simulink library "aerolibwind2"  (Simulink 6.0)
values from neighbouring files (symbols this model uses):
  s = aeroliblist    [asbhelp.m]
undefined symbols (not defined in the file or in its folder): F, ft, Light, m, MIL
libraries: aerolibconvert x11, aerolibwind2 x10, simulink x5, aerolibwindfilters x4, aerolibutil x2
settings Model: Creator=sgage  LastModifiedBy=sgage  ExtModeAutoUpdateStatusClock=off

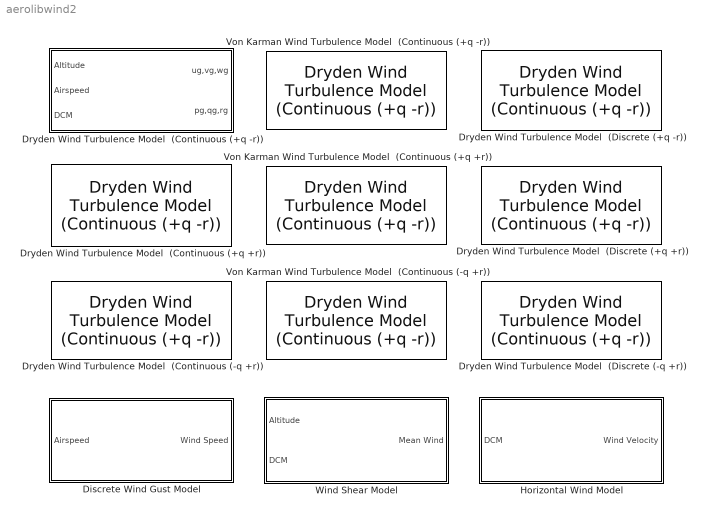
== system aerolibwind2 ==
  Discrete Wind Gust Model : Subsystem  mask(Discrete Wind Gust Model){units=Metric (MKS), Gx=on, Gy=on, Gz=on, t_0=5, d_m=[120 120 80], v_m=[3.5 3.5 3.0]}
      mask prompts: Gx "Gust in u-axis"; Gy "Gust in v-axis"; Gz "Gust in w-axis"; t_0 "Gust start time (sec):"; d_m "Gust length [dx dy dz] (m):"; v_m "Gust amplitude [ug vg wg] (m/s):"
      mask help: Generate a discrete wind gust. The gust profile takes the '1-cosine' form.
      mask init:
      | [ports] = aeroicon('aeroblkwindgust2','icon');
      | [x y highstr lowstr maxy miny] = aeroimage('wind','Discrete Gust');
      mask Help: web(asbhelp);
      mask StyleString: popup(Metric (MKS)|English (Velocity in ft/s)|English (Velocity in kts)),checkbox,checkbox,checkbox,edit,edit,edit
      mask Display:
      | port_label(ports(1).type,ports(1).port,ports(1).txt,'texmode','on');
      | port_label(ports(2).type,ports(2).port,ports(2).txt,'texmode','on');
      | plot(x,y)
      | text(0.5,miny-0.05,lowstr,'HorizontalAlignment','center')
  Dryden Wind Turbulence Model  (Continuous (+q +r)) : aerolibwind2/Dryden Wind Turbulence Model  (Continuous (+q -r))  units=Metric (MKS)  spec=MIL-F-8785C  model=Continuous Dryden (+q +r)  W20=15  Wdeg=0  TurbProb=10^-2 - Light  L_high=533.4  Wingspan=10  ts=0.1  Seed=[23341 23342 23343 23344]  T_on=on
  Dryden Wind Turbulence Model  (Continuous (+q -r)) : Subsystem  mask(Wind Turbulence Model){units=Metric (MKS), spec=MIL-F-8785C, model=Continuous Dryden (+q -r), W20=15, Wdeg=0, TurbProb=10^-2 - Light, L_high=533.4, Wingspan=10, ts=0.1, Seed=[23341 23342 23343 23344], T_on=on}
      mask prompts: spec "Specification:"; model "Model type:"; W20 "Wind speed at 6 m defines the low-altitude intensity (m/s):"; Wdeg "Wind direction at 6 m (degrees clockwise from north):"; TurbProb "Probability of exceedance of high-altitude intensity:"; L_high "Scale length at medium/high altitudes (m):"; Wingspan "Wingspan (m):"; ts "Band limited noise sample time (sec):"; Seed "Noise seeds [ug vg wg pg]:"; T_on "Turbulence on"
      mask help:
      | Generate atmospheric turbulence. White noise is passed through a filter to give the turbulence the specified velocity spectra.
      |
      | Medium/high altitude scale lengths from the specifications are 762 m (2500 ft) for Von Karman turbulence and 533.4 m (1750 ft) for Dryden turbulence.
      mask init:
      | index = strfind(model,' ');
      | disp1 = model(1:index(1)-1);
      | disp2 = model(index(1)+1:index(end-1)-1);
      | disp3 = model(index(end-1)+1:end);
      | 
      | [x y highstr lowstr maxy miny] = aeroimage('wind',[disp2 '\n' disp3],disp1);
      | 
      | h_vec = [.5 1.75 3.75 7.5 15 25 35 45 55 65 75 80]*1000;% feet
      | sigma_vec(1,:) = [3.2 2.2 1.5 zeros(1,9)]; % ft/sec
      | sigma_vec(2,:) = [4.2 3.6 3.3 1.6 zeros(1,8)];
      | sigma_vec(3,:) = [6.6 6.9 7.4 6.7 4.6 2.7 0.4 zeros(1,5)];
      | sigma_vec(4,:) = [8.6 9.6 10.6 10.1 8.0 6.6 5.0 4.2 2.7 zeros(1,3)];
      | sigma_vec(5,:) = [11.8 13.0 16.0 15.1 11.6 9.7 8.1 8.2 7.9 4.9 3.2 2.1];
      | sigma_vec(6,:) = [15.6 17.6 23.0 23.6 22.1 20.0 16.0 15.1 12.1 7.9 6.2 5.1];
      | sigma_vec(7,:) = [18.7 21.5 28.4 30.2 30.7 31.0 25.2 23.1 17.5 10.7 8.4 7.2];
      | max_height_low = 1000;
      | if strcmp(spec,'MIL-F-8785C')
      |     min_height_high = 2000;
      | else
      | 	min_height_high = 1750;
      | end
      | [ports] = aeroicon('aeroblkwindturb2','icon');
      | 
      | dt=ts;
      mask Help: web(asbhelp('Dryden Wind Turbulence Model (Continuous)'));
      mask StyleString: popup(Metric (MKS)|English (Velocity in ft/s)|English (Velocity in kts)),popup(MIL-F-8785C|MIL-HDBK-1797),popup(Continuous Von Karman (+q -r)|Continuous Von Karman (+q +r)|Continuous Von Karman (-q +r)|Continuous Dryden (+q -r)|Continuous Dryden (+q +r)|Continuous Dryden (-q +r)|Discrete Dryden (+q -r)|Discrete Dryden (+q +r)|Discrete Dryden (-q +r)),edit,edit,popup(2x10^-1|10^-1|10^-2 - Light |10^-3 - Moderate|10^-4|10^-5 - Severe|10^-6),edit,edit,edit,edit,checkbox
      mask CallbackString: ||aeroicon('aeroblkwindturb2');||||||||
      mask Display:
      | port_label(ports(1).type,ports(1).port,ports(1).txt,'texmode','on');
      | port_label(ports(2).type,ports(2).port,ports(2).txt,'texmode','on');
      | port_label(ports(3).type,ports(3).port,ports(3).txt,'texmode','on');
      | port_label(ports(4).type,ports(4).port,ports(4).txt,'texmode','on');
      | port_label(ports(5).type,ports(5).port,ports(5).txt,'texmode','on');
      | plot(x,y)
      | text(0.5,miny-0.05,lowstr,'HorizontalAlignment','center','verticalalignment','top')
      | text(0.5,maxy,highstr,'HorizontalAlignment','center','verticalalignment','bottom')
  Dryden Wind Turbulence Model  (Continuous (-q +r)) : aerolibwind2/Dryden Wind Turbulence Model  (Continuous (+q -r))  units=Metric (MKS)  spec=MIL-F-8785C  model=Continuous Dryden (-q +r)  W20=15  Wdeg=0  TurbProb=10^-2 - Light  L_high=533.4  Wingspan=10  ts=0.1  Seed=[23341 23342 23343 23344]  T_on=on
  Dryden Wind Turbulence Model  (Discrete (+q +r)) : aerolibwind2/Dryden Wind Turbulence Model  (Continuous (+q -r))  units=Metric (MKS)  spec=MIL-F-8785C  model=Discrete Dryden (+q +r)  W20=15  Wdeg=0  TurbProb=10^-2 - Light  L_high=533.4  Wingspan=10  ts=0.1  Seed=[23341 23342 23343 23344]  T_on=on
  Dryden Wind Turbulence Model  (Discrete (+q -r)) : aerolibwind2/Dryden Wind Turbulence Model  (Continuous (+q -r))  units=Metric (MKS)  spec=MIL-F-8785C  model=Discrete Dryden (+q -r)  W20=15  Wdeg=0  TurbProb=10^-2 - Light  L_high=533.4  Wingspan=10  ts=0.1  Seed=[23341 23342 23343 23344]  T_on=on
  Dryden Wind Turbulence Model  (Discrete (-q +r)) : aerolibwind2/Dryden Wind Turbulence Model  (Continuous (+q -r))  units=Metric (MKS)  spec=MIL-F-8785C  model=Discrete Dryden (-q +r)  W20=15  Wdeg=0  TurbProb=10^-2 - Light  L_high=533.4  Wingspan=10  ts=0.1  Seed=[23341 23342 23343 23344]  T_on=on
  Horizontal Wind Model : Subsystem  mask(Horizontal Wind Model){units=Metric (MKS), Vw_source=Internal, Vwind=15, W_source=Internal, Wdeg=0}
      mask prompts: Vw_source "Wind speed source:"; Vwind "Wind speed at altitude (m/s):"; W_source "Wind direction source:"; Wdeg "Wind direction at altitude (degrees clockwise from north):"
      mask help: Transform horizontal wind (north and east components) into body coordinates given wind speed, wind direction and direction cosine matrix (DCM).
      mask init:
      | [ports]=aeroicon('aeroblkhwind','icon');
      | [x y highstr lowstr maxy miny] = aeroimage('wind','Horizontal');
      mask Help: web(asbhelp);
      mask StyleString: popup(Metric (MKS)|English (Velocity in ft/s)|English (Velocity in kts)),popup(Internal|External),edit,popup(Internal|External),edit
      mask CallbackString: |aeroicon('aeroblkhwind');||aeroicon('aeroblkhwind');|
      mask Display:
      | port_label(ports(1).type,ports(1).port,ports(1).txt,'texmode','on');
      | port_label(ports(2).type,ports(2).port,ports(2).txt,'texmode','on');
      | port_label(ports(3).type,ports(3).port,ports(3).txt,'texmode','on');
      | port_label(ports(4).type,ports(4).port,ports(4).txt,'texmode','on');
      | plot(x,y)
      | text(0.5,miny-0.05,lowstr,'HorizontalAlignment','center')
  Von Karman Wind Turbulence Model  (Continuous (+q +r)) : aerolibwind2/Dryden Wind Turbulence Model  (Continuous (+q -r))  units=Metric (MKS)  spec=MIL-F-8785C  model=Continuous Von Karman (+q +r)  W20=15  Wdeg=0  TurbProb=10^-2 - Light  L_high=762  Wingspan=10  ts=0.1  Seed=[23341 23342 23343 23344]  T_on=on
  Von Karman Wind Turbulence Model  (Continuous (+q -r)) : aerolibwind2/Dryden Wind Turbulence Model  (Continuous (+q -r))  units=Metric (MKS)  spec=MIL-F-8785C  model=Continuous Von Karman (+q -r)  W20=15  Wdeg=0  TurbProb=10^-2 - Light  L_high=762  Wingspan=10  ts=0.1  Seed=[23341 23342 23343 23344]  T_on=on
  Von Karman Wind Turbulence Model  (Continuous (-q +r)) : aerolibwind2/Dryden Wind Turbulence Model  (Continuous (+q -r))  units=Metric (MKS)  spec=MIL-F-8785C  model=Continuous Von Karman (-q +r)  W20=15  Wdeg=0  TurbProb=10^-2 - Light  L_high=762  Wingspan=10  ts=0.1  Seed=[23341 23342 23343 23344]  T_on=on
  Wind Shear Model : Subsystem  mask(Wind Shear Model){units=Metric (MKS), phase=Category C - Terminal Flight Phase, W_20=15, Wdeg=0}
      mask prompts: phase "Flight phase:"; W_20 "Wind speed at 6 m altitude (m/s):"; Wdeg "Wind direction at 6 m altitude (degrees clockwise from north):"
      mask help: Calculate the wind shear from conditions measured at a height of 6 meters (20 feet) above the ground.
      mask init:
      | if phase == 1
      | 	z0 = 0.15;
      | else
      | 	z0=2.0;
      | end
      | [ports]=aeroicon('aeroblkwindshear2','icon');
      | [x y highstr lowstr maxy miny] = aeroimage('wind','Shear');
      mask Help: web(asbhelp);
      mask StyleString: popup(Metric (MKS)|English (Velocity in ft/s)|English (Velocity in kts)),popup(Category C - Terminal Flight Phase|Other),edit,edit
      mask Display:
      | port_label(ports(1).type,ports(1).port,ports(1).txt,'texmode','on');
      | port_label(ports(2).type,ports(2).port,ports(2).txt,'texmode','on');
      | port_label(ports(3).type,ports(3).port,ports(3).txt,'texmode','on');
      | plot(x,y)
      | text(0.5,miny-0.05,lowstr,'HorizontalAlignment','center')

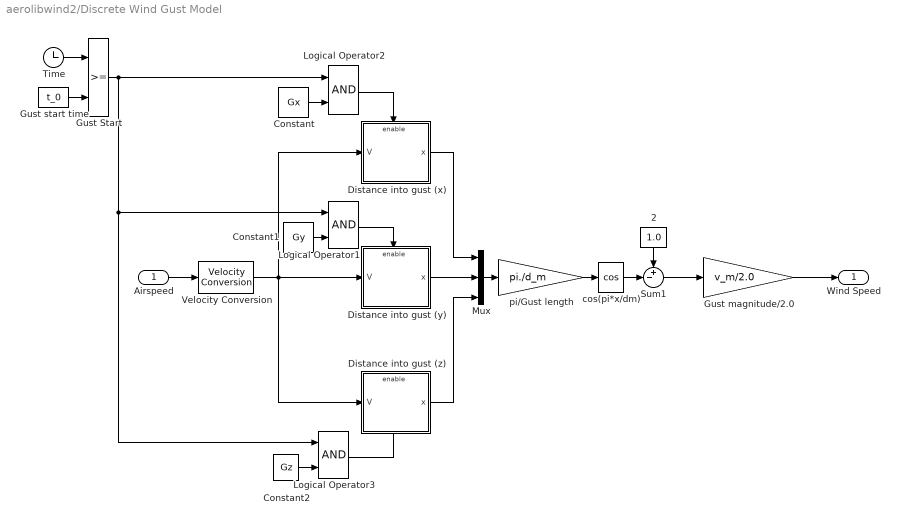
== system aerolibwind2/Discrete Wind Gust Model ==
  Airspeed : Inport  DataType=double
  2 : Constant  Orientation=down  Value=1.0
  Constant : Constant  Value=Gx
  Constant1 : Constant  Value=Gy
  Constant2 : Constant  Value=Gz
  Distance into gust (x) : Subsystem  TreatAsAtomicUnit=on  mask{d_m=d_m(1)}
      mask prompts: d_m "Gust length d:"
  Distance into gust (y) : Subsystem  TreatAsAtomicUnit=on  mask{d_m=d_m(2)}
      mask prompts: d_m "Gust length d:"
  Distance into gust (z) : Subsystem  TreatAsAtomicUnit=on  mask{d_m=d_m(3)}
      mask prompts: d_m "Gust length d:"
  Gust Start : RelationalOperator  LogicOutDataTypeMode=Specify via dialog  LogicDataType=float('double')  InputSameDT=on
  Gust magnitude/2.0 : Gain  Gain=v_m/2.0  SaturateOnIntegerOverflow=on
  Gust start time : Constant  Value=t_0
  Logical Operator1 : Logic  AllPortsSameDT=off
  Logical Operator2 : Logic  AllPortsSameDT=off
  Logical Operator3 : Logic  AllPortsSameDT=off
  Mux : Mux  Inputs=3
  Sum1 : Sum  Inputs=+-|  SaturateOnIntegerOverflow=on  InputSameDT=on
  Time : Clock
      settings: Decimation=10
  Velocity Conversion : aerolibconvert/Velocity Conversion  IU=m/s  OU=m/s
  cos(pi*x/dm) : Trigonometry  Operator=cos
  pi/Gust length : Gain  Gain=pi./d_m  SaturateOnIntegerOverflow=on
  Wind Speed : Outport
  wires:
  pi/Gust length/1 -> cos(pi*x/dm)/1
  2/1 -> Sum1/1
  Sum1/1 -> Gust magnitude/2.0/1
  cos(pi*x/dm)/1 -> Sum1/2
  Gust magnitude/2.0/1 -> Wind Speed/1
  Time/1 -> Gust Start/1
  Gust start time/1 -> Gust Start/2
  Distance into gust (y)/1(x) -> Mux/2
  Distance into gust (z)/1(x) -> Mux/3
  Mux/1 -> pi/Gust length/1
  Logical Operator3/1 -> Distance into gust (z)/Enable
  Constant2/1 -> Logical Operator3/2
  Logical Operator1/1 -> Distance into gust (y)/Enable
  Constant1/1 -> Logical Operator1/2
  Logical Operator2/1 -> Distance into gust (x)/Enable
  Airspeed/1 -> Velocity Conversion/1
  Gust Start/1 -> Logical Operator1/1, Logical Operator3/1, Logical Operator2/1
  Constant/1 -> Logical Operator2/2
  Distance into gust (x)/1(x) -> Mux/1
  Velocity Conversion/1 -> Distance into gust (y)/1(V), Distance into gust (x)/1(V), Distance into gust (z)/1(V)

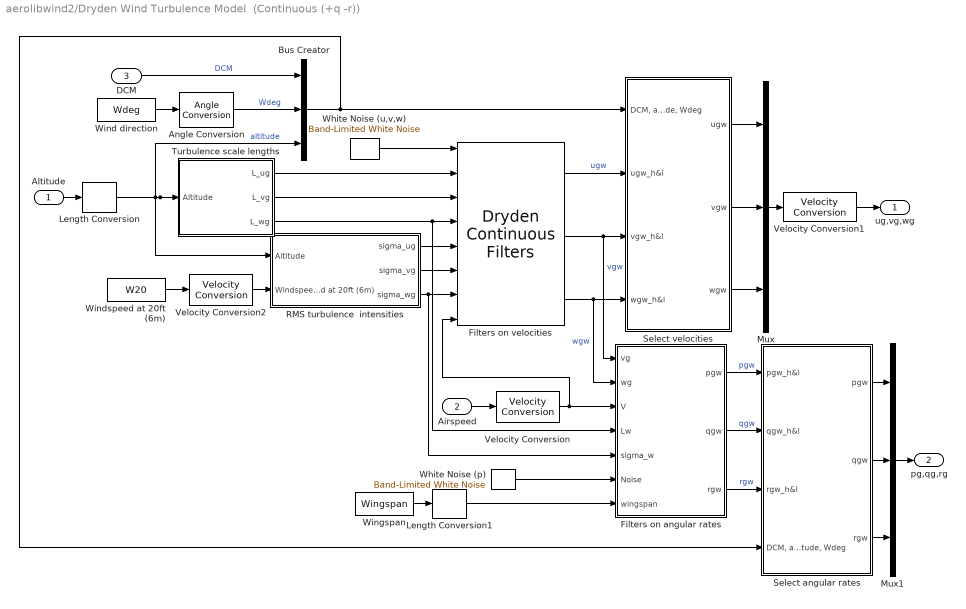
== system aerolibwind2/Dryden Wind Turbulence Model  (Continuous (+q -r)) ==
  Altitude : Inport
  Airspeed : Inport  Port=2
  DCM : Inport  Port=3
  Angle Conversion : aerolibconvert/Angle Conversion  IU=deg  OU=rad
  Bus Creator : BusCreator  Inputs=3
  Filters on angular rates : Subsystem
      mask Type: Angular Rates
  Filters on velocities : aerolibwindfilters/Dryden Continuous Filters
  Length Conversion : aerolibconvert/Length Conversion  IU=m  OU=ft
  Length Conversion1 : aerolibconvert/Length Conversion  IU=m  OU=ft
  Mux : Mux  Inputs=3
  Mux1 : Mux  Inputs=3
  RMS turbulence  intensities : Subsystem
  Select angular rates : Subsystem
  Select velocities : Subsystem
  Turbulence scale lengths : Subsystem
  Velocity Conversion : aerolibconvert/Velocity Conversion  IU=m/s  OU=ft/s
  Velocity Conversion1 : aerolibconvert/Velocity Conversion  IU=ft/s  OU=m/s
  Velocity Conversion2 : aerolibconvert/Velocity Conversion  IU=m/s  OU=ft/s
  White Noise (p) : simulink/Sources/Band-Limited White Noise  Cov=pi  Ts=ts  seed=Seed(4)
  White Noise (u,v,w) : simulink/Sources/Band-Limited White Noise  Cov=[1 1 1]*pi  Ts=ts  seed=Seed(1:3)
  Wind direction : Constant  Value=Wdeg
  Windspeed at 20ft (6m) : Constant  Value=W20
  Wingspan : Constant  Value=Wingspan
  ug,vg,wg : Outport
  pg,qg,rg : Outport  Port=2
  wires:
  Turbulence scale lengths/2(L_vg) -> Filters on velocities/3
  Length Conversion/1 -> RMS turbulence  intensities/1(Altitude), Bus Creator/3, Turbulence scale lengths/1(Altitude)  "altitude"
  White Noise (p)/1 -> Filters on angular rates/6(Noise)
  White Noise (u,v,w)/1 -> Filters on velocities/1
  Velocity Conversion1/1 -> ug,vg,wg/1
  Altitude/1 -> Length Conversion/1
  Airspeed/1 -> Velocity Conversion/1
  Velocity Conversion/1 -> Filters on velocities/8, Filters on angular rates/3(V)
  Turbulence scale lengths/1(L_ug) -> Filters on velocities/2
  Turbulence scale lengths/3(L_wg) -> Filters on velocities/4, Filters on angular rates/4(Lw)
  RMS turbulence  intensities/3(sigma_wg) -> Filters on velocities/7, Filters on angular rates/5(sigma_w)
  Mux/1 -> Velocity Conversion1/1
  Mux1/1 -> pg,qg,rg/1
  Filters on angular rates/1(pgw) -> Select angular rates/1(pgw_h&l)  "pgw"
  Filters on angular rates/2(qgw) -> Select angular rates/2(qgw_h&l)  "qgw"
  Filters on angular rates/3(rgw) -> Select angular rates/3(rgw_h&l)  "rgw"
  Filters on velocities/1 -> Select velocities/2(ugw_h&l)  "ugw"
  RMS turbulence  intensities/1("sigma_ug ") -> Filters on velocities/5
  Filters on velocities/2 -> Select velocities/3(vgw_h&l), Filters on angular rates/1(vg)  "vgw"
  Filters on velocities/3 -> Select velocities/4(wgw_h&l), Filters on angular rates/2(wg)  "wgw"
  RMS turbulence  intensities/2(sigma_vg) -> Filters on velocities/6
  Windspeed at 20ft (6m)/1 -> Velocity Conversion2/1
  Velocity Conversion2/1 -> RMS turbulence  intensities/2(Windspeed at 20ft (6m))
  Wind direction/1 -> Angle Conversion/1
  Select velocities/1(ugw) -> Mux/1
  Select velocities/2(vgw) -> Mux/2
  Select velocities/3(wgw) -> Mux/3
  Select angular rates/1(pgw) -> Mux1/1
  Select angular rates/2(qgw) -> Mux1/2
  Select angular rates/3(rgw) -> Mux1/3
  Angle Conversion/1 -> Bus Creator/2  "Wdeg"
  DCM/1 -> Bus Creator/1  "DCM"
  Bus Creator/1 -> Select velocities/1("DCM, altitude, Wdeg"), Select angular rates/4("DCM, altitude, Wdeg")
  Length Conversion1/1 -> Filters on angular rates/7(wingspan)
  Wingspan/1 -> Length Conversion1/1

== system aerolibwind2/Horizontal Wind Model ==
  DCM : Inport
  " " : Gain  Gain=-1  SaturateOnIntegerOverflow=on
  Angle Conversion : aerolibconvert/Angle Conversion  IU=deg  OU=rad
  Mux : Mux  Inputs=3
  Product1 : Product  SaturateOnIntegerOverflow=on  InputSameDT=on
  SinCos : aerolibutil/SinCos
  Transform from Inertial to Body axes : Product  Inputs=**  Multiplication=Matrix(*)  SaturateOnIntegerOverflow=on  InputSameDT=on
  Wdeg1 : Constant  Value=0
  Wind Direction : Constant  Value=Wdeg
  Wind Speed : Constant  Value=Vwind
  Wind Velocity : Outport
  wires:
  Wind Direction/1 -> Angle Conversion/1
  Wind Speed/1 -> Product1/1
  Transform from Inertial to Body axes/1 -> Wind Velocity/1
  DCM/1 -> Transform from Inertial to Body axes/1
  SinCos/2 -> Mux/1  "Wx"
  SinCos/1 -> Mux/2  "Wy"
  Angle Conversion/1 -> SinCos/1
  Wdeg1/1 -> Mux/3  "Wz"
  Mux/1 -> " "/1
  Product1/1 -> Transform from Inertial to Body axes/2
  " "/1 -> Product1/2

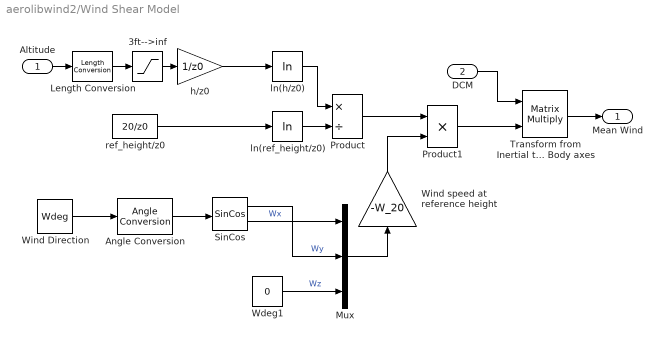
== system aerolibwind2/Wind Shear Model ==
  Altitude : Inport
  DCM : Inport  Port=2
  3ft-->inf : Saturate  UpperLimit=inf  LowerLimit=3
  Angle Conversion : aerolibconvert/Angle Conversion  IU=deg  OU=rad
  Length Conversion : aerolibconvert/Length Conversion  IU=m  OU=ft
  Mux : Mux  Inputs=3
  Product : Product  Inputs=*/  SaturateOnIntegerOverflow=on  InputSameDT=on
  Product1 : Product  SaturateOnIntegerOverflow=on  InputSameDT=on
  SinCos : aerolibutil/SinCos
  Transform from Inertial to Body axes : Product  Inputs=**  Multiplication=Matrix(*)  SaturateOnIntegerOverflow=on  InputSameDT=on
  Wdeg1 : Constant  Value=0
  Wind Direction : Constant  Value=Wdeg
  Wind speed at reference height : Gain  Orientation=up  Gain=-W_20  SaturateOnIntegerOverflow=on
  h/z0 : Gain  Gain=1/z0  SaturateOnIntegerOverflow=on
  ln(h/z0) : Math  Operator=log  SaturateOnIntegerOverflow=on
  ln(ref_height/z0) : Math  Operator=log  SaturateOnIntegerOverflow=on
  ref_height/z0 : Constant  Value=20/z0
  Mean Wind : Outport
  wires:
  Altitude/1 -> Length Conversion/1
  Product/1 -> Product1/1
  ln(ref_height/z0)/1 -> Product/2
  ln(h/z0)/1 -> Product/1
  ref_height/z0/1 -> ln(ref_height/z0)/1
  h/z0/1 -> ln(h/z0)/1
  3ft-->inf/1 -> h/z0/1
  Transform from Inertial to Body axes/1 -> Mean Wind/1
  Wind Direction/1 -> Angle Conversion/1
  SinCos/2 -> Mux/1  "Wx"
  SinCos/1 -> Mux/2  "Wy"
  Wdeg1/1 -> Mux/3  "Wz"
  Mux/1 -> Wind speed at reference height/1
  Product1/1 -> Transform from Inertial to Body axes/2
  DCM/1 -> Transform from Inertial to Body axes/1
  Wind speed at reference height/1 -> Product1/2
  Length Conversion/1 -> 3ft-->inf/1
  Angle Conversion/1 -> SinCos/1

== system aerolibwind2/Discrete Wind Gust Model/Distance into gust (x) ==
  V : Inport
  Enable : EnablePort  StatesWhenEnabling=reset
  Distance into Gust (x) (Limited to gust length d) : Integrator  LimitOutput=on  UpperSaturationLimit=d_m  LowerSaturationLimit=0
  x : Outport  InitialOutput=[0]
  wires:
  V/1 -> Distance into Gust (x) (Limited to gust length d)/1
  Distance into Gust (x) (Limited to gust length d)/1 -> x/1

== system aerolibwind2/Discrete Wind Gust Model/Distance into gust (y) ==
  V : Inport
  Enable : EnablePort  StatesWhenEnabling=reset
  "Distance into Gust (x) (Limited to gust length d) " : Integrator  LimitOutput=on  UpperSaturationLimit=d_m  LowerSaturationLimit=0
  x : Outport  InitialOutput=[0]
  wires:
  V/1 -> "Distance into Gust (x) (Limited to gust length d) "/1
  "Distance into Gust (x) (Limited to gust length d) "/1 -> x/1

== system aerolibwind2/Discrete Wind Gust Model/Distance into gust (z) ==
  V : Inport
  Enable : EnablePort  StatesWhenEnabling=reset
  "Distance into Gust (x) (Limited to gust length d) " : Integrator  LimitOutput=on  UpperSaturationLimit=d_m  LowerSaturationLimit=0
  x : Outport  InitialOutput=[0]
  wires:
  "Distance into Gust (x) (Limited to gust length d) "/1 -> x/1
  V/1 -> "Distance into Gust (x) (Limited to gust length d) "/1

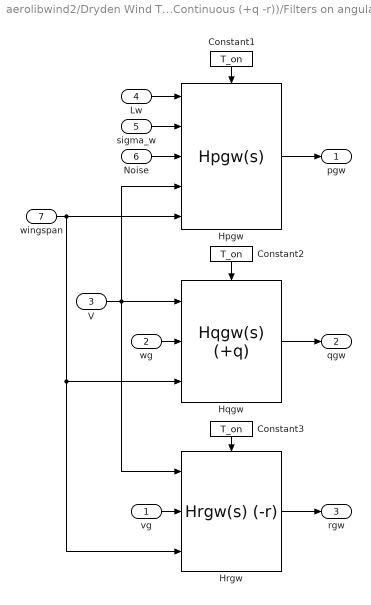
== system aerolibwind2/Dryden Wind Turbulence Model  (Continuous (+q -r))/Filters on angular rates ==
  vg : Inport
  wg : Inport  Port=2
  V : Inport  Port=3
  Lw : Inport  Port=4
  sigma_w : Inport  Port=5
  Noise : Inport  Port=6
  wingspan : Inport  Port=7
  Constant1 : Constant  Orientation=down  Value=T_on
  Constant2 : Constant  Orientation=down  Value=T_on
  Constant3 : Constant  Orientation=down  Value=T_on
  Hpgw : aerolibwindfilters/Hpgw(s)
  Hqgw : aerolibwindfilters/Hqgw(s) (+q)
  Hrgw : aerolibwindfilters/Hrgw(s) (-r)
  pgw : Outport  InitialOutput=0
  qgw : Outport  Port=2  InitialOutput=0
  rgw : Outport  Port=3  InitialOutput=0
  wires:
  wingspan/1 -> Hpgw/5, Hrgw/3, Hqgw/3
  vg/1 -> Hrgw/2
  Hrgw/1 -> rgw/1
  Hqgw/1 -> qgw/1
  wg/1 -> Hqgw/2
  Hpgw/1 -> pgw/1
  V/1 -> Hrgw/1, Hqgw/1, Hpgw/4
  sigma_w/1 -> Hpgw/2
  Lw/1 -> Hpgw/1
  Noise/1 -> Hpgw/3
  Constant1/1 -> Hpgw/Enable
  Constant2/1 -> Hqgw/Enable
  Constant3/1 -> Hrgw/Enable

== system aerolibwind2/Dryden Wind Turbulence Model  (Continuous (+q -r))/RMS turbulence  intensities ==
  Altitude : Inport
  Windspeed at 20ft (6m) : Inport  Port=2
  High Altitude Intensity : Subsystem
  Low Altitude Intensity : Subsystem
  Mux1 : Mux  Inputs=2
  Mux2 : Mux  Inputs=2
  "sigma_ug " : Outport
  sigma_vg : Outport  Port=2
  sigma_wg : Outport  Port=3
  wires:
  Altitude/1 -> Low Altitude Intensity/2(h), High Altitude Intensity/1(h)
  Low Altitude Intensity/1(sigma_ug sigma_vg) -> Mux2/1
  Low Altitude Intensity/2(sigma_wg) -> Mux1/1
  Mux1/1 -> sigma_wg/1  "sigmawg"
  High Altitude Intensity/1(sigma_ug sigma_vg sigma_wg) -> Mux1/2, Mux2/2
  Windspeed at 20ft (6m)/1 -> Low Altitude Intensity/1(Windspeed  at 20ft (6m))
  Mux2/1 -> "sigma_ug "/1, sigma_vg/1  "sigmaug"

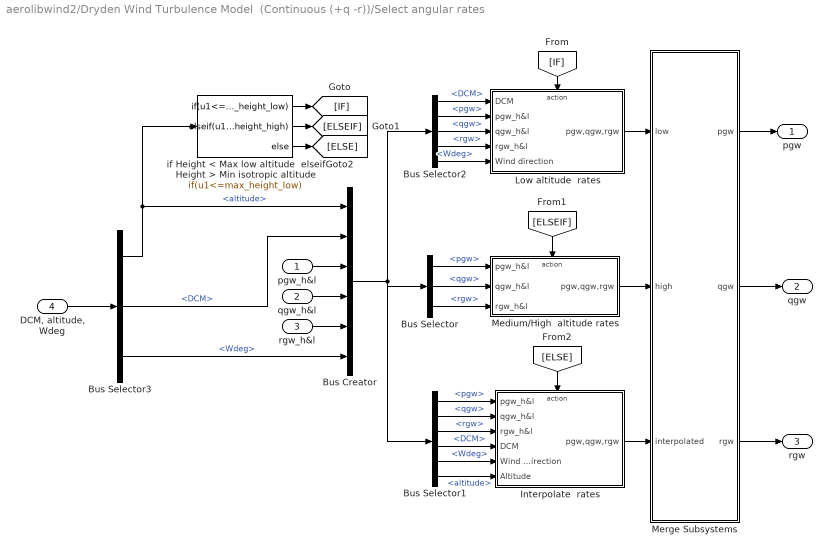
== system aerolibwind2/Dryden Wind Turbulence Model  (Continuous (+q -r))/Select angular rates ==
  pgw_h&l : Inport
  qgw_h&l : Inport  Port=2
  rgw_h&l : Inport  Port=3
  "DCM, altitude, Wdeg" : Inport  Port=4
  Bus Creator : BusCreator  Inputs=6
  Bus Selector : BusSelector  OutputSignals=pgw,qgw,rgw
  Bus Selector1 : BusSelector  OutputSignals=pgw,qgw,rgw,DCM,Wdeg,altitude
  Bus Selector2 : BusSelector  OutputSignals=DCM,pgw,qgw,rgw,Wdeg
  Bus Selector3 : BusSelector  OutputSignals=altitude,DCM,Wdeg
  Interpolate  rates : Subsystem  TreatAsAtomicUnit=on
  Low altitude  rates : Subsystem  TreatAsAtomicUnit=on
  Medium/High  altitude rates : Subsystem  TreatAsAtomicUnit=on
  Merge Subsystems : Subsystem
  "if Height < Max low altitude  elseif Height > Min isotropic altitude " : If  IfExpression=u1<=max_height_low  ElseIfExpressions=u1>=min_height_high
  pgw : Outport  InitialOutput=0
  qgw : Outport  Port=2  InitialOutput=0
  rgw : Outport  Port=3  InitialOutput=0
  wires:
  Low altitude  rates/1(pgw,qgw,rgw) -> Merge Subsystems/1(low)
  Medium/High  altitude rates/1(pgw,qgw,rgw) -> Merge Subsystems/2(high)
  "if Height < Max low altitude  elseif Height > Min isotropic altitude "/3 -> [ELSE]
  [ELSE] -> Interpolate  rates/Action
  [ELSEIF] -> Medium/High  altitude rates/Action
  "if Height < Max low altitude  elseif Height > Min isotropic altitude "/2 -> [ELSEIF]
  [IF] -> Low altitude  rates/Action
  "if Height < Max low altitude  elseif Height > Min isotropic altitude "/1 -> [IF]
  Bus Selector1/5 -> Interpolate  rates/5(Wind direction)  "<Wdeg>"
  Bus Selector2/5 -> Low altitude  rates/5(Wind direction)  "<Wdeg>"
  Bus Selector3/3 -> Bus Creator/6  "<Wdeg>"
  Interpolate  rates/1(pgw,qgw,rgw) -> Merge Subsystems/3(interpolated)
  Merge Subsystems/3(rgw) -> rgw/1
  Merge Subsystems/2(qgw) -> qgw/1
  Merge Subsystems/1(pgw) -> pgw/1
  Bus Selector/3 -> Medium/High  altitude rates/3(rgw_h&l)  "<rgw>"
  Bus Selector/2 -> Medium/High  altitude rates/2(qgw_h&l)  "<qgw>"
  Bus Selector/1 -> Medium/High  altitude rates/1(pgw_h&l)  "<pgw>"
  Bus Selector2/4 -> Low altitude  rates/4(rgw_h&l)  "<rgw>"
  Bus Selector2/3 -> Low altitude  rates/3(qgw_h&l)  "<qgw>"
  Bus Selector2/2 -> Low altitude  rates/2(pgw_h&l)  "<pgw>"
  Bus Selector2/1 -> Low altitude  rates/1(DCM)  "<DCM>"
  Bus Selector1/6 -> Interpolate  rates/6(Altitude)  "<altitude>"
  Bus Selector1/4 -> Interpolate  rates/4(DCM)  "<DCM>"
  Bus Selector1/3 -> Interpolate  rates/3(rgw_h&l)  "<rgw>"
  Bus Selector1/2 -> Interpolate  rates/2(qgw_h&l)  "<qgw>"
  Bus Selector1/1 -> Interpolate  rates/1(pgw_h&l)  "<pgw>"
  rgw_h&l/1 -> Bus Creator/5
  qgw_h&l/1 -> Bus Creator/4
  pgw_h&l/1 -> Bus Creator/3
  Bus Selector3/2 -> Bus Creator/2  "<DCM>"
  Bus Creator/1 -> Bus Selector2/1, Bus Selector/1, Bus Selector1/1
  Bus Selector3/1 -> "if Height < Max low altitude  elseif Height > Min isotropic altitude "/1, Bus Creator/1  "<altitude>"
  "DCM, altitude, Wdeg"/1 -> Bus Selector3/1

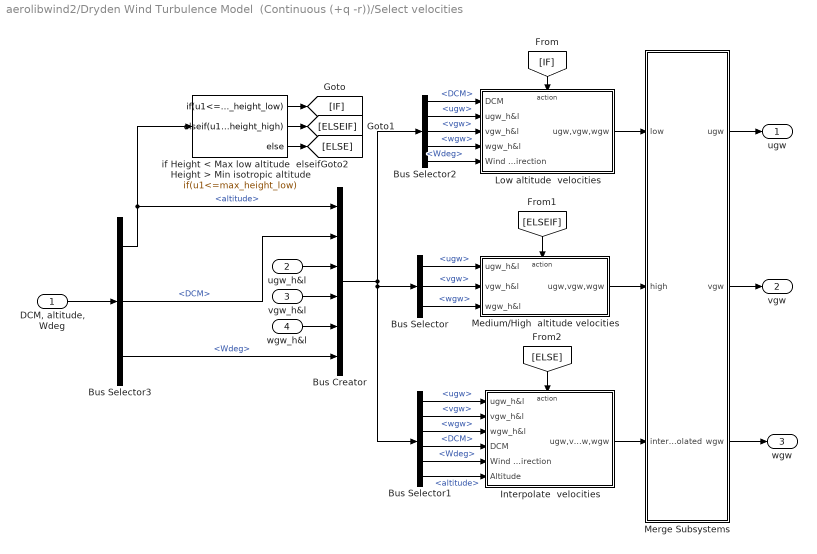
== system aerolibwind2/Dryden Wind Turbulence Model  (Continuous (+q -r))/Select velocities ==
  "DCM, altitude, Wdeg" : Inport
  ugw_h&l : Inport  Port=2
  vgw_h&l : Inport  Port=3
  wgw_h&l : Inport  Port=4
  Bus Creator : BusCreator  Inputs=6
  Bus Selector : BusSelector  OutputSignals=ugw,vgw,wgw
  Bus Selector1 : BusSelector  OutputSignals=ugw,vgw,wgw,DCM,Wdeg,altitude
  Bus Selector2 : BusSelector  OutputSignals=DCM,ugw,vgw,wgw,Wdeg
  Bus Selector3 : BusSelector  OutputSignals=altitude,DCM,Wdeg
  Interpolate  velocities : Subsystem  TreatAsAtomicUnit=on
  Low altitude  velocities : Subsystem  TreatAsAtomicUnit=on
  Medium/High  altitude velocities : Subsystem  TreatAsAtomicUnit=on
  Merge Subsystems : Subsystem
  "if Height < Max low altitude  elseif Height > Min isotropic altitude " : If  IfExpression=u1<=max_height_low  ElseIfExpressions=u1>=min_height_high
  ugw : Outport  InitialOutput=0
  vgw : Outport  Port=2  InitialOutput=0
  wgw : Outport  Port=3  InitialOutput=0
  wires:
  Bus Selector3/1 -> "if Height < Max low altitude  elseif Height > Min isotropic altitude "/1, Bus Creator/1  "<altitude>"
  Bus Creator/1 -> Bus Selector1/1, Bus Selector/1, Bus Selector2/1
  Bus Selector3/2 -> Bus Creator/2  "<DCM>"
  ugw_h&l/1 -> Bus Creator/3
  vgw_h&l/1 -> Bus Creator/4
  wgw_h&l/1 -> Bus Creator/5
  Bus Selector1/1 -> Interpolate  velocities/1(ugw_h&l)  "<ugw>"
  Bus Selector1/2 -> Interpolate  velocities/2(vgw_h&l)  "<vgw>"
  Bus Selector1/3 -> Interpolate  velocities/3(wgw_h&l)  "<wgw>"
  Bus Selector1/4 -> Interpolate  velocities/4(DCM)  "<DCM>"
  Bus Selector2/1 -> Low altitude  velocities/1(DCM)  "<DCM>"
  Bus Selector2/2 -> Low altitude  velocities/2(ugw_h&l)  "<ugw>"
  Bus Selector2/3 -> Low altitude  velocities/3(vgw_h&l)  "<vgw>"
  Bus Selector2/4 -> Low altitude  velocities/4(wgw_h&l)  "<wgw>"
  Bus Selector/1 -> Medium/High  altitude velocities/1(ugw_h&l)  "<ugw>"
  Bus Selector/2 -> Medium/High  altitude velocities/2(vgw_h&l)  "<vgw>"
  Bus Selector/3 -> Medium/High  altitude velocities/3(wgw_h&l)  "<wgw>"
  Merge Subsystems/1(ugw) -> ugw/1
  Merge Subsystems/2(vgw) -> vgw/1
  Merge Subsystems/3(wgw) -> wgw/1
  Interpolate  velocities/1(ugw,vgw,wgw) -> Merge Subsystems/3(interpolated)
  Bus Selector3/3 -> Bus Creator/6  "<Wdeg>"
  Bus Selector2/5 -> Low altitude  velocities/5(Wind direction)  "<Wdeg>"
  Bus Selector1/5 -> Interpolate  velocities/5(Wind direction)  "<Wdeg>"
  "if Height < Max low altitude  elseif Height > Min isotropic altitude "/1 -> [IF]
  [IF] -> Low altitude  velocities/Action
  "if Height < Max low altitude  elseif Height > Min isotropic altitude "/2 -> [ELSEIF]
  [ELSEIF] -> Medium/High  altitude velocities/Action
  [ELSE] -> Interpolate  velocities/Action
  "if Height < Max low altitude  elseif Height > Min isotropic altitude "/3 -> [ELSE]
  Medium/High  altitude velocities/1(ugw,vgw,wgw) -> Merge Subsystems/2(high)
  Low altitude  velocities/1(ugw,vgw,wgw) -> Merge Subsystems/1(low)
  Bus Selector1/6 -> Interpolate  velocities/6(Altitude)  "<altitude>"
  "DCM, altitude, Wdeg"/1 -> Bus Selector3/1

== system aerolibwind2/Dryden Wind Turbulence Model  (Continuous (+q -r))/Turbulence scale lengths ==
  Altitude : Inport
  Low altitude scale length : Subsystem
  Lv : Gain  SaturateOnIntegerOverflow=on
  Lw : Gain  SaturateOnIntegerOverflow=on
  Medium/High altitude scale length : Subsystem
  Mux : Mux  Inputs=2
  Mux1 : Mux  Inputs=2
  L_ug : Outport
  L_vg : Outport  Port=2
  L_wg : Outport  Port=3
  wires:
  Medium/High altitude scale length/1(L_ug L_vg L_wg) -> Mux/2, Mux1/2
  Low altitude scale length/2(L_wg) -> Mux/1
  Low altitude scale length/1(L_ug L_vg) -> Mux1/1
  Mux1/1 -> L_ug/1, Lv/1  "Lug"
  Mux/1 -> Lw/1  "Lwg"
  Altitude/1 -> Low altitude scale length/1(h)
  Lw/1 -> L_wg/1
  Lv/1 -> L_vg/1

== system aerolibwind2/Dryden Wind Turbulence Model  (Continuous (+q -r))/RMS turbulence  intensities/High Altitude Intensity ==
  h : Inport
  Medium/High Altitude Intensity : simulink/Lookup Tables/Interpolation (n-D) using PreLookup  numDimsPopupSelect=2  explicitNumDims=2  table=sigma_vec'  interpMethod=Linear  extrapMethod=Linear  rangeErrorMode=None  NumSelectionDims=0
  PreLook-Up Index Search  (altitude) : simulink/Lookup Tables/PreLookup Index Search  bpData=h_vec  searchMode=Binary Search  cacheBpFlag=on  outputFlag=off  IndexDataType=uint32  extrapMode=Clip to Range  rangeErrorMode=None
  PreLook-Up Index Search  (prob of exceed) : simulink/Lookup Tables/PreLookup Index Search  bpData=[1:7]  searchMode=Binary Search  cacheBpFlag=on  outputFlag=off  IndexDataType=uint32  extrapMode=Linear Extrapolation  rangeErrorMode=None
  Probability of  Exceedance : Constant  Value=TurbProb
  sigma_ug sigma_vg sigma_wg : Outport  InitialOutput=0
  wires:
  Probability of  Exceedance/1 -> PreLook-Up Index Search  (prob of exceed)/1
  Medium/High Altitude Intensity/1 -> sigma_ug sigma_vg sigma_wg/1
  h/1 -> PreLook-Up Index Search  (altitude)/1
  PreLook-Up Index Search  (altitude)/1 -> Medium/High Altitude Intensity/1
  PreLook-Up Index Search  (prob of exceed)/1 -> Medium/High Altitude Intensity/2

== system aerolibwind2/Dryden Wind Turbulence Model  (Continuous (+q -r))/RMS turbulence  intensities/Low Altitude Intensity ==
  Windspeed  at 20ft (6m) : Inport
  h : Inport  Port=2
  Limit Height h<1000ft : Saturate  UpperLimit=max_height_low  LowerLimit=0
  Low Altitude Intensity : Fcn  Expr=1/(0.177+0.000823*u(1))^0.4
  "sigma_ug, sigma_vg" : Product  SaturateOnIntegerOverflow=on  InputSameDT=on
  "sigma_wg " : Gain  Gain=0.1  SaturateOnIntegerOverflow=on
  sigma_ug sigma_vg : Outport  InitialOutput=0
  sigma_wg : Outport  Port=2  InitialOutput=0
  wires:
  Limit Height h<1000ft/1 -> Low Altitude Intensity/1
  Windspeed  at 20ft (6m)/1 -> "sigma_wg "/1
  "sigma_wg "/1 -> "sigma_ug, sigma_vg"/2, sigma_wg/1
  Low Altitude Intensity/1 -> "sigma_ug, sigma_vg"/1
  h/1 -> Limit Height h<1000ft/1
  "sigma_ug, sigma_vg"/1 -> sigma_ug sigma_vg/1

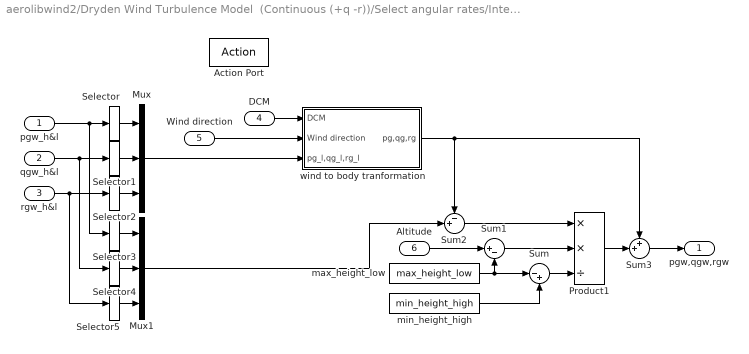
== system aerolibwind2/Dryden Wind Turbulence Model  (Continuous (+q -r))/Select angular rates/Interpolate  rates ==
  pgw_h&l : Inport
  qgw_h&l : Inport  Port=2
  rgw_h&l : Inport  Port=3
  DCM : Inport  Port=4
  Wind direction : Inport  Port=5
  Altitude : Inport  Port=6
  Action Port : ActionPort
  Mux : Mux  Inputs=3
  Mux1 : Mux  Inputs=3
  Product1 : Product  Inputs=**/  SaturateOnIntegerOverflow=on
  Selector : Selector  InputPortWidth=2
  Selector1 : Selector  InputPortWidth=2
  Selector2 : Selector  InputPortWidth=2
  Selector3 : Selector  Elements=2  InputPortWidth=2
  Selector4 : Selector  Elements=2  InputPortWidth=2
  Selector5 : Selector  Elements=2  InputPortWidth=2
  Sum : Sum  Inputs=|-+  SaturateOnIntegerOverflow=on
  Sum1 : Sum  Inputs=|+-  SaturateOnIntegerOverflow=on
  Sum2 : Sum  Inputs=-+|  SaturateOnIntegerOverflow=on
  Sum3 : Sum  Inputs=++|  SaturateOnIntegerOverflow=on
  max_height_low : Constant  Value=max_height_low
  min_height_high : Constant  Value=min_height_high
  wind to body tranformation : Subsystem
  pgw,qgw,rgw : Outport  InitialOutput=0
  wires:
  Selector2/1 -> Mux/3
  Selector1/1 -> Mux/2
  Selector/1 -> Mux/1
  rgw_h&l/1 -> Selector2/1, Selector5/1
  qgw_h&l/1 -> Selector1/1, Selector4/1
  pgw_h&l/1 -> Selector3/1, Selector/1
  Selector5/1 -> Mux1/3
  Selector4/1 -> Mux1/2
  Selector3/1 -> Mux1/1
  Wind direction/1 -> wind to body tranformation/2(Wind direction)
  max_height_low/1 -> Sum/1, Sum1/2
  min_height_high/1 -> Sum/2
  Altitude/1 -> Sum1/1
  Sum/1 -> Product1/3
  Sum1/1 -> Product1/2
  Sum2/1 -> Product1/1
  Mux1/1 -> Sum2/2
  Product1/1 -> Sum3/2
  Sum3/1 -> pgw,qgw,rgw/1
  wind to body tranformation/1(pg,qg,rg) -> Sum2/1, Sum3/1
  DCM/1 -> wind to body tranformation/1(DCM)
  Mux/1 -> wind to body tranformation/3(pg_l,qg_l,rg_l)

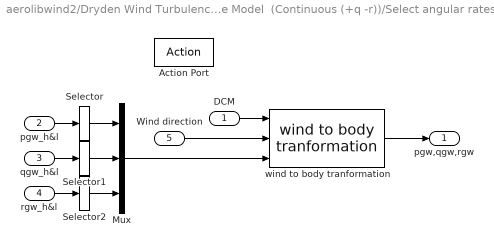
== system aerolibwind2/Dryden Wind Turbulence Model  (Continuous (+q -r))/Select angular rates/Low altitude  rates ==
  DCM : Inport
  pgw_h&l : Inport  Port=2
  qgw_h&l : Inport  Port=3
  rgw_h&l : Inport  Port=4
  Wind direction : Inport  Port=5
  Action Port : ActionPort
  Mux : Mux  Inputs=3
  Selector : Selector  InputPortWidth=2
  Selector1 : Selector  InputPortWidth=2
  Selector2 : Selector  InputPortWidth=2
  wind to body tranformation : aerolibwind2/Dryden Wind Turbulence Model  (Continuous (+q -r))/Select angular rates/Interpolate  rates/wind to body tranformation  SimViewingDevice=off  DataTypeOverride=UseLocalSettings  MinMaxOverflowLogging=UseLocalSettings
      settings: Permissions=ReadWrite  RTWFcnNameOpts=Auto  RTWFileNameOpts=Auto
  pgw,qgw,rgw : Outport  InitialOutput=0
  wires:
  Wind direction/1 -> wind to body tranformation/2
  wind to body tranformation/1 -> pgw,qgw,rgw/1
  Mux/1 -> wind to body tranformation/3
  Selector2/1 -> Mux/3
  Selector1/1 -> Mux/2
  Selector/1 -> Mux/1
  rgw_h&l/1 -> Selector2/1
  qgw_h&l/1 -> Selector1/1
  pgw_h&l/1 -> Selector/1
  DCM/1 -> wind to body tranformation/1

== system aerolibwind2/Dryden Wind Turbulence Model  (Continuous (+q -r))/Select angular rates/Medium/High  altitude rates ==
  pgw_h&l : Inport
  qgw_h&l : Inport  Port=2
  rgw_h&l : Inport  Port=3
  Action Port : ActionPort
  Gain : Gain  SaturateOnIntegerOverflow=on
  Mux : Mux  Inputs=3
  Selector3 : Selector  Elements=[ 2 4 6]  InputPortWidth=6
  pgw,qgw,rgw : Outport  InitialOutput=0
  wires:
  Mux/1 -> Selector3/1
  rgw_h&l/1 -> Mux/3
  qgw_h&l/1 -> Mux/2
  pgw_h&l/1 -> Mux/1
  Selector3/1 -> Gain/1
  Gain/1 -> pgw,qgw,rgw/1

== system aerolibwind2/Dryden Wind Turbulence Model  (Continuous (+q -r))/Select angular rates/Merge Subsystems ==
  low : Inport
  high : Inport  Port=2
  interpolated : Inport  Port=3
  Demux : Demux  Outputs=3
  Merge : Merge  Inputs=3
  pgw : Outport
  qgw : Outport  Port=2
  rgw : Outport  Port=3
  wires:
  Merge/1 -> Demux/1
  Demux/1 -> pgw/1
  Demux/3 -> rgw/1
  Demux/2 -> qgw/1
  interpolated/1 -> Merge/3
  high/1 -> Merge/2
  low/1 -> Merge/1

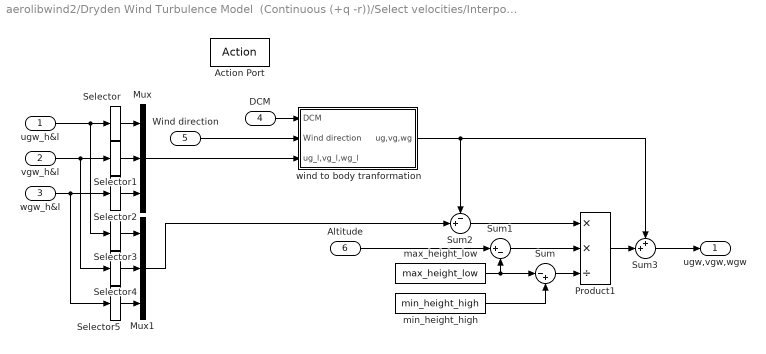
== system aerolibwind2/Dryden Wind Turbulence Model  (Continuous (+q -r))/Select velocities/Interpolate  velocities ==
  ugw_h&l : Inport
  vgw_h&l : Inport  Port=2
  wgw_h&l : Inport  Port=3
  DCM : Inport  Port=4
  Wind direction : Inport  Port=5
  Altitude : Inport  Port=6
  Action Port : ActionPort
  Mux : Mux  Inputs=3
  Mux1 : Mux  Inputs=3
  Product1 : Product  Inputs=**/  SaturateOnIntegerOverflow=on
  Selector : Selector  InputPortWidth=2
  Selector1 : Selector  InputPortWidth=2
  Selector2 : Selector  InputPortWidth=2
  Selector3 : Selector  Elements=2  InputPortWidth=2
  Selector4 : Selector  Elements=2  InputPortWidth=2
  Selector5 : Selector  Elements=2  InputPortWidth=2
  Sum : Sum  Inputs=|-+  SaturateOnIntegerOverflow=on
  Sum1 : Sum  Inputs=|+-  SaturateOnIntegerOverflow=on
  Sum2 : Sum  Inputs=-+|  SaturateOnIntegerOverflow=on
  Sum3 : Sum  Inputs=++|  SaturateOnIntegerOverflow=on
  max_height_low : Constant  Value=max_height_low
  min_height_high : Constant  Value=min_height_high
  wind to body tranformation : Subsystem
  ugw,vgw,wgw : Outport  InitialOutput=0
  wires:
  Selector2/1 -> Mux/3
  Selector1/1 -> Mux/2
  Selector/1 -> Mux/1
  wgw_h&l/1 -> Selector2/1, Selector5/1
  vgw_h&l/1 -> Selector1/1, Selector4/1
  ugw_h&l/1 -> Selector3/1, Selector/1
  Selector5/1 -> Mux1/3
  Selector4/1 -> Mux1/2
  Selector3/1 -> Mux1/1
  max_height_low/1 -> Sum/1, Sum1/2
  min_height_high/1 -> Sum/2
  Altitude/1 -> Sum1/1
  Sum/1 -> Product1/3
  Sum1/1 -> Product1/2
  Sum2/1 -> Product1/1
  Mux1/1 -> Sum2/2
  Product1/1 -> Sum3/2
  Sum3/1 -> ugw,vgw,wgw/1
  wind to body tranformation/1(ug,vg,wg) -> Sum2/1, Sum3/1
  DCM/1 -> wind to body tranformation/1(DCM)
  Wind direction/1 -> wind to body tranformation/2(Wind direction)
  Mux/1 -> wind to body tranformation/3(ug_l,vg_l,wg_l)

== system aerolibwind2/Dryden Wind Turbulence Model  (Continuous (+q -r))/Select velocities/Low altitude  velocities ==
  DCM : Inport
  ugw_h&l : Inport  Port=2
  vgw_h&l : Inport  Port=3
  wgw_h&l : Inport  Port=4
  Wind direction : Inport  Port=5
  Action Port : ActionPort
  Mux : Mux  Inputs=3
  Selector : Selector  InputPortWidth=2
  Selector1 : Selector  InputPortWidth=2
  Selector2 : Selector  InputPortWidth=2
  wind to body tranformation : aerolibwind2/Dryden Wind Turbulence Model  (Continuous (+q -r))/Select velocities/Interpolate  velocities/wind to body tranformation  SimViewingDevice=off  DataTypeOverride=UseLocalSettings  MinMaxOverflowLogging=UseLocalSettings
      settings: Permissions=ReadWrite  RTWFcnNameOpts=Auto  RTWFileNameOpts=Auto
  ugw,vgw,wgw : Outport  InitialOutput=0
  wires:
  ugw_h&l/1 -> Selector/1
  vgw_h&l/1 -> Selector1/1
  wgw_h&l/1 -> Selector2/1
  Selector/1 -> Mux/1
  Selector1/1 -> Mux/2
  DCM/1 -> wind to body tranformation/1
  Wind direction/1 -> wind to body tranformation/2
  wind to body tranformation/1 -> ugw,vgw,wgw/1
  Selector2/1 -> Mux/3
  Mux/1 -> wind to body tranformation/3

== system aerolibwind2/Dryden Wind Turbulence Model  (Continuous (+q -r))/Select velocities/Medium/High  altitude velocities ==
  ugw_h&l : Inport
  vgw_h&l : Inport  Port=2
  wgw_h&l : Inport  Port=3
  Action Port : ActionPort
  Gain : Gain  SaturateOnIntegerOverflow=on
  Mux : Mux  Inputs=3
  Selector3 : Selector  Elements=[ 2 4 6]  InputPortWidth=6
  ugw,vgw,wgw : Outport  InitialOutput=0
  wires:
  ugw_h&l/1 -> Mux/1
  wgw_h&l/1 -> Mux/3
  Mux/1 -> Selector3/1
  Selector3/1 -> Gain/1
  Gain/1 -> ugw,vgw,wgw/1
  vgw_h&l/1 -> Mux/2

== system aerolibwind2/Dryden Wind Turbulence Model  (Continuous (+q -r))/Select velocities/Merge Subsystems ==
  low : Inport
  high : Inport  Port=2
  interpolated : Inport  Port=3
  Demux : Demux  Outputs=3
  Merge : Merge  Inputs=3
  ugw : Outport
  vgw : Outport  Port=2
  wgw : Outport  Port=3
  wires:
  low/1 -> Merge/1
  high/1 -> Merge/2
  interpolated/1 -> Merge/3
  Demux/2 -> vgw/1
  Demux/3 -> wgw/1
  Demux/1 -> ugw/1
  Merge/1 -> Demux/1

== system aerolibwind2/Dryden Wind Turbulence Model  (Continuous (+q -r))/Turbulence scale lengths/Low altitude scale length ==
  h : Inport
  Limit Function 10ft to 1000ft : Saturate  UpperLimit=max_height_low  LowerLimit=10
  Low Altitude Scale Length : Fcn  Expr=u(1)/(0.177+0.000823*u(1))^1.2
  L_ug L_vg : Outport  InitialOutput=0
  L_wg : Outport  Port=2  InitialOutput=0
  wires:
  Limit Function 10ft to 1000ft/1 -> Low Altitude Scale Length/1, L_wg/1
  Low Altitude Scale Length/1 -> L_ug L_vg/1
  h/1 -> Limit Function 10ft to 1000ft/1

== system aerolibwind2/Dryden Wind Turbulence Model  (Continuous (+q -r))/Turbulence scale lengths/Medium/High altitude scale length ==
  Length Conversion : aerolibconvert/Length Conversion  IU=m  OU=ft
  Medium/High Altitude : Constant  Value=L_high
  L_ug L_vg L_wg : Outport  InitialOutput=0
  wires:
  Length Conversion/1 -> L_ug L_vg L_wg/1
  Medium/High Altitude/1 -> Length Conversion/1

== system aerolibwind2/Dryden Wind Turbulence Model  (Continuous (+q -r))/Select angular rates/Interpolate  rates/wind to body tranformation ==
  DCM : Inport
  Wind direction : Inport  Port=2
  pg_l,qg_l,rg_l : Inport  Port=3
  Demux : Demux  Outputs=3
  Mux2 : Mux  Inputs=3
  Product : Product  Multiplication=Matrix(*)  SaturateOnIntegerOverflow=on
  convert to earth coords : Subsystem
  pg,qg,rg : Outport
  wires:
  pg_l,qg_l,rg_l/1 -> Demux/1
  Product/1 -> pg,qg,rg/1
  Demux/3 -> Mux2/3
  Demux/2 -> convert to earth coords/3(qg_l)
  Demux/1 -> convert to earth coords/2(pg_l)
  Mux2/1 -> Product/2
  convert to earth coords/2(qg) -> Mux2/2
  convert to earth coords/1(pg) -> Mux2/1
  Wind direction/1 -> convert to earth coords/1(Wind direction)
  DCM/1 -> Product/1

== system aerolibwind2/Dryden Wind Turbulence Model  (Continuous (+q -r))/Select velocities/Interpolate  velocities/wind to body tranformation ==
  DCM : Inport
  Wind direction : Inport  Port=2
  ug_l,vg_l,wg_l : Inport  Port=3
  Demux : Demux  Outputs=3
  Mux2 : Mux  Inputs=3
  Product : Product  Multiplication=Matrix(*)  SaturateOnIntegerOverflow=on
  convert to earth coords : Subsystem
  ug,vg,wg : Outport
  wires:
  DCM/1 -> Product/1
  Wind direction/1 -> convert to earth coords/1(Wind direction)
  convert to earth coords/1(ug) -> Mux2/1
  convert to earth coords/2(vg) -> Mux2/2
  Mux2/1 -> Product/2
  Demux/1 -> convert to earth coords/2(ug_l)
  Demux/2 -> convert to earth coords/3(vg_l)
  Demux/3 -> Mux2/3
  Product/1 -> ug,vg,wg/1
  ug_l,vg_l,wg_l/1 -> Demux/1

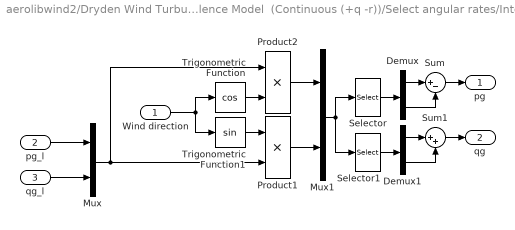
== system aerolibwind2/Dryden Wind Turbulence Model  (Continuous (+q -r))/Select angular rates/Interpolate  rates/wind to body tranformation/convert to earth coords ==
  Wind direction : Inport
  pg_l : Inport  Port=2
  qg_l : Inport  Port=3
  Demux : Demux  Outputs=2
  Demux1 : Demux  Outputs=2
  Mux : Mux  Inputs=2
  Mux1 : Mux  Inputs=2
  Product1 : Product  SaturateOnIntegerOverflow=on  InputSameDT=on
  Product2 : Product  SaturateOnIntegerOverflow=on  InputSameDT=on
  Selector : Selector  Elements=[1 4]  InputPortWidth=4
  Selector1 : Selector  Elements=[2 3]  InputPortWidth=4
  Sum : Sum  Inputs=|+-  SaturateOnIntegerOverflow=on
  Sum1 : Sum  Inputs=|++  SaturateOnIntegerOverflow=on
  Trigonometric Function : Trigonometry  Operator=cos
  Trigonometric Function1 : Trigonometry
  pg : Outport
  qg : Outport  Port=2
  wires:
  Wind direction/1 -> Trigonometric Function/1, Trigonometric Function1/1
  pg_l/1 -> Mux/1
  qg_l/1 -> Mux/2
  Trigonometric Function1/1 -> Product1/1
  Mux/1 -> Product1/2, Product2/1
  Trigonometric Function/1 -> Product2/2
  Sum/1 -> pg/1
  Sum1/1 -> qg/1
  Demux/1 -> Sum/1
  Demux/2 -> Sum/2
  Demux1/1 -> Sum1/1
  Demux1/2 -> Sum1/2
  Product2/1 -> Mux1/1
  Product1/1 -> Mux1/2
  Mux1/1 -> Selector/1, Selector1/1
  Selector/1 -> Demux/1
  Selector1/1 -> Demux1/1

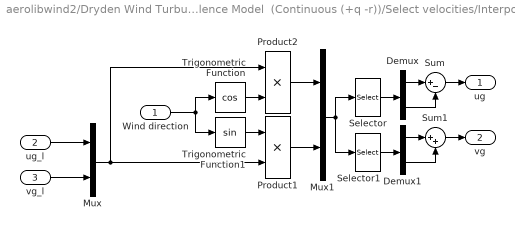
== system aerolibwind2/Dryden Wind Turbulence Model  (Continuous (+q -r))/Select velocities/Interpolate  velocities/wind to body tranformation/convert to earth coords ==
  Wind direction : Inport
  ug_l : Inport  Port=2
  vg_l : Inport  Port=3
  Demux : Demux  Outputs=2
  Demux1 : Demux  Outputs=2
  Mux : Mux  Inputs=2
  Mux1 : Mux  Inputs=2
  Product1 : Product  SaturateOnIntegerOverflow=on  InputSameDT=on
  Product2 : Product  SaturateOnIntegerOverflow=on  InputSameDT=on
  Selector : Selector  Elements=[1 4]  InputPortWidth=4
  Selector1 : Selector  Elements=[2 3]  InputPortWidth=4
  Sum : Sum  Inputs=|+-  SaturateOnIntegerOverflow=on
  Sum1 : Sum  Inputs=|++  SaturateOnIntegerOverflow=on
  Trigonometric Function : Trigonometry  Operator=cos
  Trigonometric Function1 : Trigonometry
  ug : Outport
  vg : Outport  Port=2
  wires:
  Selector1/1 -> Demux1/1
  Selector/1 -> Demux/1
  Mux1/1 -> Selector1/1, Selector/1
  Product1/1 -> Mux1/2
  Product2/1 -> Mux1/1
  Demux1/2 -> Sum1/2
  Demux1/1 -> Sum1/1
  Demux/2 -> Sum/2
  Demux/1 -> Sum/1
  Sum1/1 -> vg/1
  Sum/1 -> ug/1
  Trigonometric Function/1 -> Product2/2
  Mux/1 -> Product2/1, Product1/2
  Trigonometric Function1/1 -> Product1/1
  vg_l/1 -> Mux/2
  ug_l/1 -> Mux/1
  Wind direction/1 -> Trigonometric Function1/1, Trigonometric Function/1
